simulink model "task5_constraint_mpc"  (R2017b)
settings: Solver=VariableStepAuto  StartTime=0.0  StopTime=60  RelTol=1e-3
values from neighbouring files (symbols this model uses):
  A = [1 1; 2 2]    [test.m]    (also in testfile.m = [-k(1)/2 * xe(1)^(-0.5),   0)
  alpha = [alpha1; alpha2]    [OAC_LA_Ass2.m]    (also in testfile.m)
  beta = [beta1; beta2]    [OAC_LA_Ass2.m]    (also in testfile.m)
  Cd = lin_dsys.C    [OAC_LA_Ass2.m]    (also in test.m = [1 4])
  F = [F;F_loop]    [Task4_Funcs.m]    (also in matrixen_david.mat = [0.0192211007699 0.0377055868389 0.0554746314453 0.072548866; test.m = [])
  Fx = [Fx;Fx_loop]    [Task5_Funcs.m]    (also in test.m)
  G = [G; G_loop]    [Task4_Funcs.m]    (also in matrixen_david.mat = [0.00453058966741 0.0178906696229 0.0397402020478 0.06974893; test.m = [])
  gamma = [gamma1; gamma2]    [OAC_LA_Ass2.m]    (also in testfile.m)
  Gx = [Gx; Gx_loop]    [Task5_Funcs.m]
  h = evalin('base','h')    [MPC_function.m]    (also in MPC_softcon_function.m; OAC_LA_Ass2.m = [h01; h02]; testfile.m = [h01; h02])
  h02 = 10.53    [OAC_LA_Ass2.m]    (also in testfile.m)
  k = [k1; k2]    [OAC_LA_Ass2.m]    (also in testfile.m)
  n = size(Ad,1)    [OAC_LA_Ass2.m]    (also in testfile.m)
  Ts = 0.5    [OAC_LA_Ass2.m]    (also in testfile.m)
  u_eq = evalin('base','u_eq')    [MPC_softcon_function.m]    (also in Task1_Funcs.m = [double(S.u1_eq); 0])
  u_lower_limit = evalin('base','u_lower_limit')    [MPC_softcon_function.m]    (also in OAC_LA_Ass2.m = 0)
  u_upper_limit = evalin('base','u_upper_limit')    [MPC_softcon_function.m]    (also in OAC_LA_Ass2.m = 5)
  x0_linear = -x_eq+h    [OAC_LA_Ass2.m]
  x_eq = evalin('base','x_eq')    [MPC_softcon_function.m]    (also in Task1_Funcs.m = [double(S.x1_eq); x2_eq])
  x_lower_limit = evalin('base','x_lower_limit')    [MPC_softcon_function.m]    (also in OAC_LA_Ass2.m = [0; 0])
  x_upper_limit = evalin('base','x_upper_limit')    [MPC_softcon_function.m]    (also in OAC_LA_Ass2.m = [20; 20])
  y_eq = 15    [OAC_LA_Ass2.m]
undefined symbols (not defined in the file or in its folder): B
settings Model: Creator=lukastotschnig  LastModifiedBy=lukastotschnig

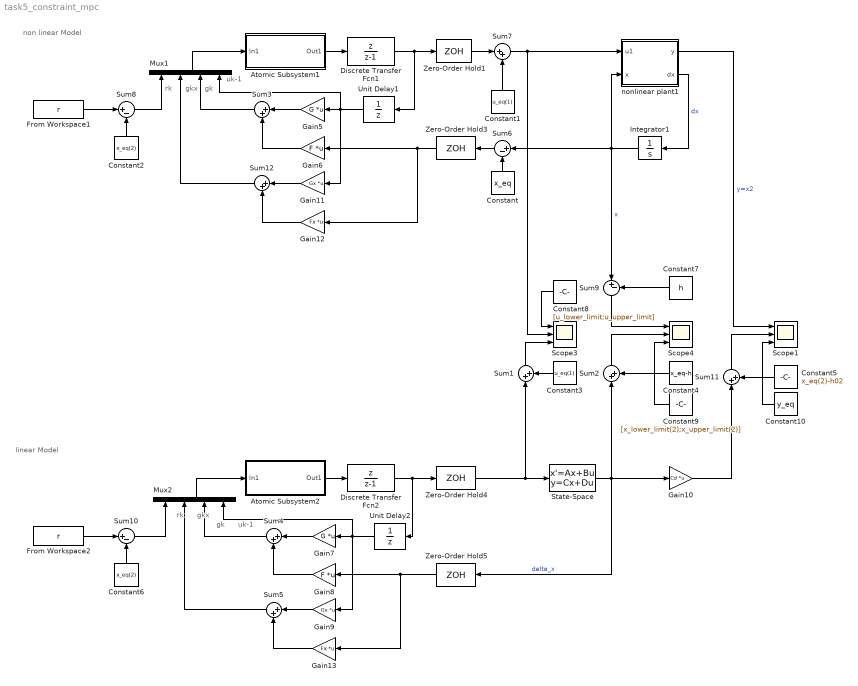
== system task5_constraint_mpc ==
  note: linear Model
  note: non linear Model
  note: gk
  note: uk-1
  note: gkx
  note: rk
  note: gk
  note: uk-1
  note: gkx
  note: rk
  Atomic Subsystem1 : Subsystem  TreatAsAtomicUnit=on  SystemSampleTime=Ts
  Atomic Subsystem2 : Subsystem  TreatAsAtomicUnit=on  SystemSampleTime=Ts
  Constant : Constant  Value=x_eq
  Constant1 : Constant  Value=u_eq(1)
  Constant10 : Constant  Value=y_eq
  Constant2 : Constant  Value=x_eq(2)
  Constant3 : Constant  Value=u_eq(1)
  Constant4 : Constant  Value=x_eq-h
  Constant5 : Constant  Value=x_eq(2)-h02
  Constant6 : Constant  Value=x_eq(2)
  Constant7 : Constant  Value=h
  Constant8 : Constant  Value=[u_lower_limit;u_upper_limit]
  Constant9 : Constant  Value=[x_lower_limit(2);x_upper_limit(2)]
  Discrete Transfer Fcn1 : DiscreteTransferFcn  Numerator=[1 0]  Denominator=[1 -1]  SampleTime=Ts
  Discrete Transfer Fcn2 : DiscreteTransferFcn  Numerator=[1 0]  Denominator=[1 -1]  SampleTime=Ts
  From Workspace1 : FromWorkspace  VariableName=r  SampleTime=0
  From Workspace2 : FromWorkspace  VariableName=r  SampleTime=0
  Gain10 : Gain  Gain=Cd  Multiplication=Matrix(K*u)
  Gain11 : Gain  Gain=Gx  Multiplication=Matrix(K*u)
  Gain12 : Gain  Gain=Fx  Multiplication=Matrix(K*u)
  Gain13 : Gain  Gain=Fx  Multiplication=Matrix(K*u)
  Gain5 : Gain  Gain=G  Multiplication=Matrix(K*u)
  Gain6 : Gain  Gain=F  Multiplication=Matrix(K*u)
  Gain7 : Gain  Gain=G  Multiplication=Matrix(K*u)
  Gain8 : Gain  Gain=F  Multiplication=Matrix(K*u)
  Gain9 : Gain  Gain=Gx  Multiplication=Matrix(K*u)
  Integrator1 : Integrator  InitialCondition=h
  Mux1 : Mux
  Mux2 : Mux
  Scope1 : Scope  NumInputPorts=3
  Scope3 : Scope  NumInputPorts=3
  Scope4 : Scope  NumInputPorts=3
  State-Space : StateSpace  A=A  B=B  C=eye(n)  D=[0;0]  InitialCondition=x0_linear
  Sum{1..5,7,11..12} (8 alike) : Sum  Inputs=|++
  Sum{6,8..10} (4 alike) : Sum  Inputs=|+-
  Unit Delay1 : UnitDelay  SampleTime=Ts
  Unit Delay2 : UnitDelay  SampleTime=Ts
  Zero-Order Hold{1,3..5} (4 alike) : ZeroOrderHold  SampleTime=Ts
  nonlinear plant1 : MATLAB Function  TreatAsAtomicUnit=on
  wires:
  Constant6/1 -> Sum10/2
  Sum7/1 -> Scope3/2, nonlinear plant1/1(u1)
  Constant2/1 -> Sum8/2
  Constant/1 -> Sum6/2
  Constant1/1 -> Sum7/2
  Constant5/1 -> Sum11/2
  nonlinear plant1/2(dx) -> Integrator1/1  "dx"
  Integrator1/1 -> nonlinear plant1/2(x), Sum6/1, Sum9/1  "x"
  nonlinear plant1/1(y) -> Scope1/1  "y=x2"
  Sum10/1 -> Mux2/1
  From Workspace2/1 -> Sum10/1
  From Workspace1/1 -> Sum8/1
  Gain10/1 -> Sum11/1
  State-Space/1 -> Gain10/1, Zero-Order Hold5/1, Sum2/1  "delta_x"
  Sum11/1 -> Scope1/2
  Gain11/1 -> Sum12/1
  Gain6/1 -> Sum3/2
  Sum12/1 -> Mux1/2
  Unit Delay1/1 -> Gain11/1, Mux1/4, Gain5/1
  Atomic Subsystem1/1(Out1) -> Discrete Transfer Fcn1/1
  Sum3/1 -> Mux1/3
  Gain5/1 -> Sum3/1
  Sum8/1 -> Mux1/1
  Gain12/1 -> Sum12/2
  Mux1/1 -> Atomic Subsystem1/1(In1)
  Gain9/1 -> Sum5/1
  Gain8/1 -> Sum4/2
  Sum5/1 -> Mux2/2
  Unit Delay2/1 -> Gain9/1, Mux2/4, Gain7/1
  Atomic Subsystem2/1(Out1) -> Discrete Transfer Fcn2/1
  Sum4/1 -> Mux2/3
  Gain7/1 -> Sum4/1
  Gain13/1 -> Sum5/2
  Mux2/1 -> Atomic Subsystem2/1(In1)
  Zero-Order Hold1/1 -> Sum7/1
  Discrete Transfer Fcn1/1 -> Unit Delay1/1, Zero-Order Hold1/1
  Sum6/1 -> Zero-Order Hold3/1
  Zero-Order Hold3/1 -> Gain12/1, Gain6/1
  Discrete Transfer Fcn2/1 -> Zero-Order Hold4/1, Unit Delay2/1
  Zero-Order Hold5/1 -> Gain13/1, Gain8/1
  Zero-Order Hold4/1 -> State-Space/1, Sum1/1
  Constant3/1 -> Sum1/2
  Sum1/1 -> Scope3/3
  Constant4/1 -> Sum2/2
  Sum2/1 -> Scope4/2
  Sum9/1 -> Scope4/1
  Constant7/1 -> Sum9/2
  Constant8/1 -> Scope3/1
  Constant9/1 -> Scope4/3
  Constant10/1 -> Scope1/3

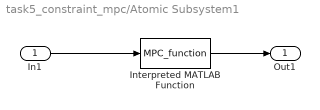
== system task5_constraint_mpc/Atomic Subsystem1 ==
  In1 : Inport
  Interpreted MATLAB Function : MATLABFcn  MATLABFcn=MPC_function
  Out1 : Outport
  wires:
  In1/1 -> Interpreted MATLAB Function/1
  Interpreted MATLAB Function/1 -> Out1/1

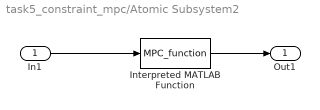
== system task5_constraint_mpc/Atomic Subsystem2 ==
  In1 : Inport
  Interpreted MATLAB Function : MATLABFcn  MATLABFcn=MPC_function
  Out1 : Outport
  wires:
  In1/1 -> Interpreted MATLAB Function/1
  Interpreted MATLAB Function/1 -> Out1/1

== matlab function task5_constraint_mpc/nonlinear plant1 ==
  data: y output; dx output; u1 input; x input; k parameter; alpha parameter; beta parameter; gamma parameter; h parameter
function [y, dx]= fcn(u1,x,k,alpha, beta, gamma,h)
    
    % calculate input quantity
    if (beta(1)+gamma(1)*u1) <= 0
        zp1 = 0;
    else
        zp1 = alpha(1) + sqrt( beta(1)+gamma(1)*u1 );
    end
    
    % nonlinear plant description
   dx1 = -k(1)*sqrt(x(1)) + zp1;
   dx2 = -k(2)*sqrt(x(2)) + k(1)*sqrt(x(1));
   
   dx = [dx1; dx2];
   y = x(2)-h(2);

end
